simulink model "batikan_cobanoglu_odev"  (R2021a)
settings: Solver=FixedStepAuto  StartTime=0.0  StopTime=0.08  FixedStep=1e-7  RelTol=1e-4
InitFcn:
  | clc;
  | clear all;
  | 
  | 
  | Kpw=1;
  | Kiw=200;
  | 
  | Kpq=0.3;
  | Kiq=200;
  | 
  | Kpd=0.5;
  | Kid=200;
  | 
  | mw=0;
  | mq=0;
  | md=0;
  | 
  | S1=1;
  | S4=0;
  | 
  | S3=0;
  | S6=1;
  | 
  | S5=0;
  | S2=1;
libraries: spsMosfetLib x6, spsCurrentMeasurementLib x3, spsSeriesRLCBranchLib x3, spsVoltageMeasurementLib x3, spsDCVoltageSourceLib x1, simulink x1, spspowerguiLib x1
Description:
  | Copyright 2008-2018 The MathWorks, Inc.
settings Model: ExtModeTrigMode=oneshot  ExtModeArmWhenConnect=off  ExtModeAutoUpdateStatusClock=off  Creator=MathWorks  LastModifiedBy=Batikan
settings SolverCC: AlgebraicLoopSolver=TrustRegion
settings DataIOCC: ExternalInput=[]  SaveFormat=Array  SignalLoggingSaveFormat=ModelDataLogs  SaveOutput=off  SaveTime=off  ReturnWorkspaceOutputs=off  SignalLoggingName=sigsOut
settings OptimizationCC: BlockReduction=off  BooleanDataType=off  ExpressionDepthLimit=2147483647  InitFltsAndDblsToZero=on  EfficientMapNaN2IntZero=off  LifeSpan=inf
settings DebuggingCC: UnderspecifiedInitializationDetection=Classic  MergeDetectMultiDrivingBlocksExec=none  CheckExecutionContextPreStartOutputMsg=on  SignalResolutionControl=TryResolveAllWithWarning  MultiTaskDSMMsg=warning  MultiTaskCondExecSysMsg=none  SigSpecEnsureSampleTimeMsg=none  FcnCallInpInsideContextMsg=warning  StateNameClashWarn=warning  SFUnexpectedBacktrackingDiag=warning  SFNoUnconditionalDefaultTransitionDiag=warning  SFMachineParentedDataDiag=warning  ArithmeticOperatorsInVariantConditions=warning
settings HardwareCC: ProdBitPerPointer=32  ProdBitPerSizeT=32  ProdBitPerPtrDiffT=32  ProdLargestAtomicFloat=None  ProdIntDivRoundTo=Undefined  ProdEndianess=Unspecified  ProdWordSize=32  ProdHWDeviceType=32-bit Generic  TargetBitPerPointer=64  TargetBitPerSizeT=64  TargetBitPerPtrDiffT=64  TargetLongLongMode=on  TargetIntDivRoundTo=Zero  TargetEndianess=LittleEndian  TargetWordSize=64  TargetHWDeviceType=MATLAB Host  ProdEqTarget=off
settings ModelReferenceCC: PropagateSignalLabelsOutOfModel=off
settings SFSimCC: SimUseLocalCustomCode=off  CustomCodeUndefinedFunction=UseInterfaceOnly
settings RTWCC: RTWUseLocalCustomCode=off
settings CodeAppCC: StateflowObjectComments=on
settings GRTTargetCC: TargetLangStandard=C89/C90 (ANSI)  CombineOutputUpdateFcns=off  GRTInterface=on
settings ConfigComp: CovMetricSettings=dw  CovSaveCumulativeToWorkspaceVar=on  CovSaveSingleToWorkspaceVar=on  CovExternalEMLEnable=off  CovSFcnEnable=off
settings SimscapeCC: SimscapeNormalizeSystem=off

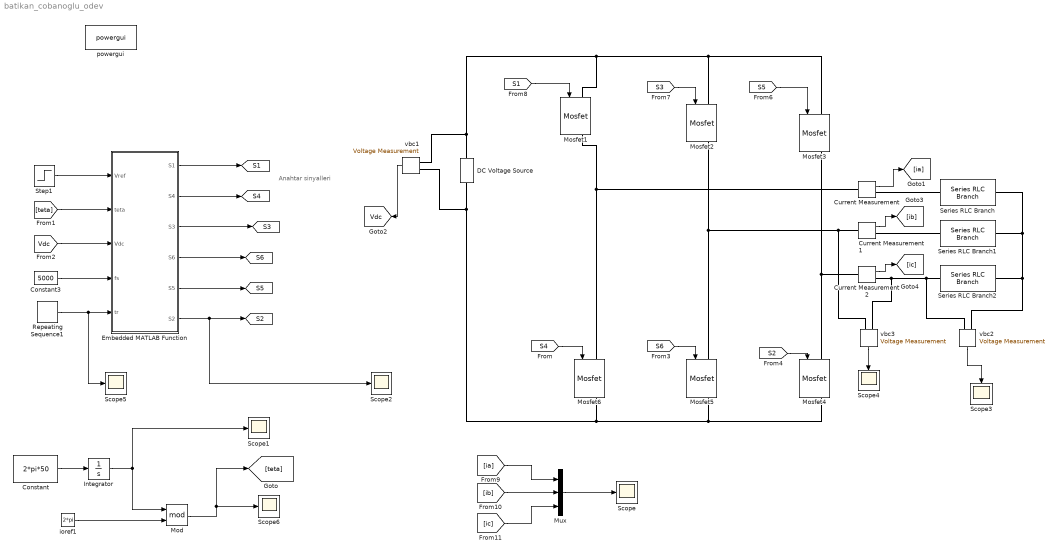
== system batikan_cobanoglu_odev ==
  note: Anahtar sinyalleri
  Constant : Constant  Value=2*pi*50
  Constant3 : Constant  Value=5000
  Current Measurement : spsCurrentMeasurementLib/Current Measurement  PhasorSimulation=off  OutputType=Complex  PSBequivalent=0
  Current Measurement1 : spsCurrentMeasurementLib/Current Measurement  PhasorSimulation=off  OutputType=Complex  PSBequivalent=0
  Current Measurement2 : spsCurrentMeasurementLib/Current Measurement  PhasorSimulation=off  OutputType=Complex  PSBequivalent=0
  DC Voltage Source : spsDCVoltageSourceLib/DC Voltage Source  Amplitude=500  Measurements=None
  Embedded MATLAB Function : MATLAB Function  TreatAsAtomicUnit=on
  Integrator : Integrator
  Mod : Math  Operator=mod  SignedPower=on  SaturateOnIntegerOverflow=on
  Mosfet{1..6} (6 alike) : spsMosfetLib/Mosfet  Ron=0.1  Lon=0  Rd=0.01  Vfd=0  IC=0  Rs=1e5  Cs=inf  Measurements=on
  Mux : Mux  Inputs=3
  Repeating Sequence1 : simulink/Sources/Repeating Sequence  rep_seq_t=[0 1e-4 2e-4]  rep_seq_y=[0 2e-4 0]
  Scope{,1..6} (7 alike) : Scope
  Series RLC Branch : spsSeriesRLCBranchLib/Series RLC Branch  LConnTagsString=__new0  RConnTagsString=__new0  BranchType=RL  Resistance=10  Inductance=10e-3  SetiL0=off  InitialCurrent=0  Capacitance=1e-6  Setx0=off  InitialVoltage=0  Measurements=None
  Series RLC Branch1 : spsSeriesRLCBranchLib/Series RLC Branch  LConnTagsString=__new0  RConnTagsString=__new0  BranchType=RL  Resistance=10  Inductance=10e-3  SetiL0=off  InitialCurrent=0  Capacitance=1e-6  Setx0=off  InitialVoltage=0  Measurements=None
  Series RLC Branch2 : spsSeriesRLCBranchLib/Series RLC Branch  LConnTagsString=__new0  RConnTagsString=__new0  BranchType=RL  Resistance=10  Inductance=10e-3  SetiL0=off  InitialCurrent=0  Capacitance=1e-6  Setx0=off  InitialVoltage=0  Measurements=None
  Step1 : Step  Time=0.04  Before=200  After=350  SampleTime=0
  ioref1 : Constant  Value=2*pi
  powergui : spspowerguiLib/powergui  SimulationMode=Discrete  SampleTime=1e-7  frequency=60  Iterations=50  frequencyindice=0  Pbase=100e6  ErrMax=1e-4  UnitsV=kV  UnitsW=MW  buscounter=0  FunctionMessages=off  echomessages=off  EnableUseOfTLC=off  CurrentSourceSwitches=off  DisableSnubberDevices=off  DisableRonSwitches=off  DisableVfSwitches=off  DisplayEquations=off  AutomaticDiscreteSolvers=off  SolverType=Tustin/Backward Euler (TBE)  Interpol=off  ExternalGateDelay=off  methode=off  Ts=100  x0status=blocks  SPID=off  SwTol=0  HookPort=off  NonlinearTolerance=1e-4  nMaxIteration=100  ContinueOnMaxIteration=off  RestoreLinks=warning  ResistiveCurrentMeasurement=off  Frange=[0:2:500]  Ylog=off  Xlog=on  ShowGrid=off  save=off  variable=ZData  structure=0  ZoomFFT=on  StartTime=0.0  cycles=1  DisplayStyle=1  fundamental=60  FreqAxis=off  MaxFrequency=1000  frequencyindicesteady=1  RmsSteady=1  display=off
  vbc1 : spsVoltageMeasurementLib/Voltage Measurement  Tag=PoWeRsYsTeMmEaSuReMeNt  PhasorSimulation=off  OutputType=Magnitude  PSBequivalent=0
  vbc2 : spsVoltageMeasurementLib/Voltage Measurement  Tag=PoWeRsYsTeMmEaSuReMeNt  PhasorSimulation=off  OutputType=Magnitude  PSBequivalent=0
  vbc3 : spsVoltageMeasurementLib/Voltage Measurement  Tag=PoWeRsYsTeMmEaSuReMeNt  PhasorSimulation=off  OutputType=Magnitude  PSBequivalent=0
  tag scope: S1=global, S2=global, S3=global, S4=global, S5=global, S6=global, Vdc=global
  wires:
  Embedded MATLAB Function/3(S3) -> [S3]
  Embedded MATLAB Function/5(S5) -> [S5]
  Repeating Sequence1/1 -> Scope5/1, Embedded MATLAB Function/5(tr)
  Constant3/1 -> Embedded MATLAB Function/4(fs)
  [Vdc] -> Embedded MATLAB Function/3(Vdc)
  Embedded MATLAB Function/1(S1) -> [S1]
  Embedded MATLAB Function/4(S6) -> [S6]
  Embedded MATLAB Function/2(S4) -> [S4]
  Embedded MATLAB Function/6(S2) -> Scope2/1, [S2]
  [teta] -> Embedded MATLAB Function/2(teta)
  vbc1/1 -> [Vdc]
  Step1/1 -> Embedded MATLAB Function/1(Vref)
  [S2] -> Mosfet4/1
  [S6] -> Mosfet5/1
  [S5] -> Mosfet3/1
  [S3] -> Mosfet2/1
  Constant/1 -> Integrator/1
  Current Measurement/1 -> [ia]
  Current Measurement1/1 -> [ib]
  Current Measurement2/1 -> [ic]
  [ia] -> Mux/1
  [ib] -> Mux/2
  [ic] -> Mux/3
  Mux/1 -> Scope/1
  ioref1/1 -> Mod/2
  Integrator/1 -> Mod/1, Scope1/1
  Mod/1 -> Scope6/1, [teta]
  vbc2/1 -> Scope3/1
  vbc3/1 -> Scope4/1
  [S1] -> Mosfet1/1
  [S4] -> Mosfet6/1
  connections:
  Mosfet5/RConn1 -- vbc1/LConn2 -- DC Voltage Source/LConn1 -- Mosfet6/RConn1 -- Mosfet4/RConn1
  Mosfet1/RConn1 -- Current Measurement/LConn1 -- Mosfet6/LConn1
  Mosfet3/RConn1 -- Current Measurement2/LConn1 -- Mosfet4/LConn1
  vbc1/LConn1 -- Mosfet1/LConn1 -- Mosfet3/LConn1 -- Mosfet2/LConn1 -- DC Voltage Source/RConn1
  Mosfet2/RConn1 -- vbc3/LConn1 -- Current Measurement1/LConn1 -- Mosfet5/LConn1
  Current Measurement/RConn1 -- Series RLC Branch/LConn1
  Current Measurement1/RConn1 -- Series RLC Branch1/LConn1
  Current Measurement2/RConn1 -- vbc3/LConn2 -- vbc2/LConn1 -- Series RLC Branch2/LConn1
  Series RLC Branch/RConn1 -- Series RLC Branch1/RConn1 -- vbc2/LConn2 -- Series RLC Branch2/RConn1

== matlab function batikan_cobanoglu_odev/Embedded MATLAB Function ==
  data: Vref input; teta input; Vdc input; S1 output; S4 output; S3 output; S6 output; S5 output; S2 output; fs input; tr input


function [S1,S4,S3,S6,S5,S2] = fcn(Vref,teta,Vdc,fs,tr)
S1=0;
S2=0;
S3=0;
S4=0;
S5=0;
S6=0;
ma=(sqrt(3)*Vref)/Vdc;
Ts=1/fs;
 if ma>1
ma=1;
 end
if(teta>0) && (teta<pi/3) %SEKTOR 1
    Ta = Ts*ma*sin(pi/3-teta);
    Tb = Ts*ma*sin(teta);
    To = Ts-Ta-Tb;
        if(tr < Ta)
            S1=1; S6=1; S2=1;
            S4=0; S3=0; S5=0;
        end
        if(tr > Ta) && (tr < Ta + Tb)
            S1=1; S3=1; S2=1;
            S4=0; S6=0; S5=0;
        end
        if(tr > Ta + Tb) && (tr < Ta + Tb + To)
            S1=1; S3=1; S5=1;
            S4=0; S6=0; S2=0;
        end
        
elseif(teta>pi/3) && (teta<2*pi/3) %SEKTOR 2 
    Ta = Ts*ma*sin((2*pi)/3-teta);
    Tb = Ts*ma*sin(teta-pi/3);
    To = Ts-Ta-Tb;
        if(tr < Ta)
            S1=1; S3=1; S2=1;
            S4=0; S6=0; S5=0;
        end
        if(tr > Ta) && (tr < Ta + Tb)
            S4=1; S3=1; S2=1;
            S1=0; S6=0; S5=0;
        end
        if(tr > Ta + Tb) && (tr < Ta + Tb + To)
            S1=1; S3=1; S5=1;
            S4=0; S6=0; S2=0;
        end
        
elseif(teta>(2*pi)/3) && (teta<(3*pi/3)) %SEKTOR 3
    Ta = Ts*ma*sin((3*pi)/3-teta);
    Tb = Ts*ma*sin(teta-(2*pi)/3);
    To = Ts-Ta-Tb;
        if(tr < Ta)
            S4=1; S3=1; S2=1;
            S1=0; S6=0; S5=0;
        end
        if(tr > Ta) && (tr < Ta + Tb)
            S4=1; S3=1; S5=1;
            S1=0; S6=0; S2=0;
        end
        if(tr > Ta + Tb) && (tr < Ta + Tb + To)
            S1=1; S3=1; S5=1;
            S4=0; S6=0; S2=0;
        end
        
elseif(teta>3*pi/3) && (teta<(4*pi)/3) %SEKTOR 4
    Ta = Ts*ma*sin((4*pi)/3-teta);
    Tb = Ts*ma*sin(teta-(3*pi)/3);
    To = Ts-Ta-Tb;
        if(tr < Ta)
            S4=1; S3=1; S5=1;
            S1=0; S6=0; S2=0;
        end
        if(tr > Ta) && (tr < Ta + Tb)
            S4=1; S6=1; S5=1;
            S1=0; S3=0; S2=0;
        end
        if(tr > Ta + Tb) && (tr < Ta + Tb + To)
            S1=1; S3=1; S5=1;
            S4=0; S6=0; S2=0;
        end
        
elseif(teta>(4*pi)/3) && (teta<(5*pi)/3) %SEKTOR 5
    Ta = Ts*ma*sin((5*pi)/3-teta);
    Tb = Ts*ma*sin(teta-(4*pi)/3);
    To = Ts-Ta-Tb;
        if(tr < Ta)
            S4=1; S6=1; S5=1;
            S1=0; S3=0; S2=0;
        end
        if(tr > Ta) && (tr < Ta + Tb)
            S1=1; S6=1; S5=1;
            S4=0; S3=0; S2=0;
        end
        if(tr > Ta + Tb) && (tr < Ta + Tb + To)
            S1=1; S3=1; S5=1;
            S4=0; S6=0; S2=0;
        end
        
elseif(teta>(5*pi)/3) && (teta<2*pi) %SEKTOR 6
    Ta = Ts*ma*sin((6*pi)/3-teta);
    Tb = Ts*ma*sin(teta-(5*pi)/3);
    To = Ts-Ta-Tb;
        if(tr < Ta)
            S1=1; S6=1; S5=1;
            S4=0; S3=0; S2=0;
        end
        if(tr > Ta) && (tr < Ta + Tb)
            S1=1; S6=1; S2=1;
            S4=0; S3=0; S5=0;
        end
        if(tr > Ta + Tb) && (tr < Ta + Tb + To)
            S1=1; S3=1; S5=1;
            S4=0; S6=0; S2=0;
        end
end
